simulink model "closed_loop2_simulink"  (R2021b)
settings: Solver=VariableStepAuto  StartTime=0.0  StopTime=15  RelTol=1e-3
values from neighbouring files (symbols this model uses):
  C = I4(1:2,:)    [open_loop.m]
  D = zeros(2,1)    [open_loop.m]
undefined symbols (not defined in the file or in its folder): A, alfa, B, beta, K, sigma_theta, sigma_x, Ts
settings Model: Creator=pieter  LastModifiedBy=pieter

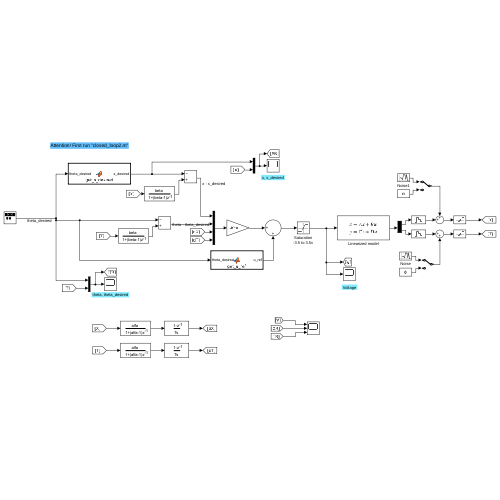
[thumbnail: Simulink's stored preview of the top-level diagram]
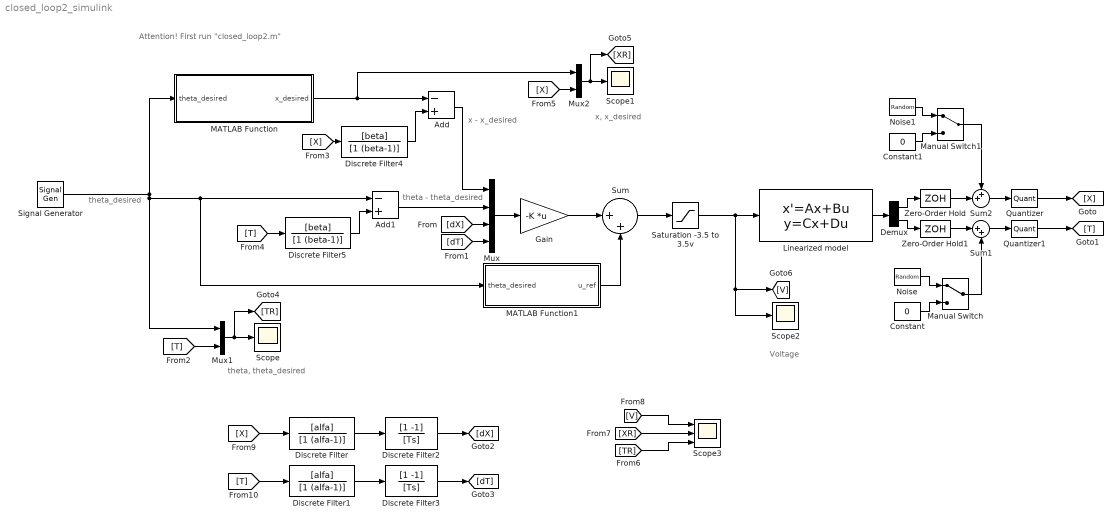
== system closed_loop2_simulink ==
  note: theta - theta_desired
  note: Attention! First run "closed_loop2.m"
  note: Voltage
  note: x - x_desired
  note: x, x_desired
  note: theta, theta_desired
  note: theta_desired
  Add : Sum  Inputs=-+
  Add1 : Sum  Inputs=-+
  Constant : Constant  Value=0
  Constant1 : Constant  Value=0
  Demux : Demux  Outputs=2
  Discrete Filter : DiscreteFilter  Numerator=[alfa]  Denominator=[1 (alfa-1)]
  Discrete Filter1 : DiscreteFilter  Numerator=[alfa]  Denominator=[1 (alfa-1)]
  Discrete Filter2 : DiscreteFilter  Numerator=[1 -1]  Denominator=[Ts]
  Discrete Filter3 : DiscreteFilter  Numerator=[1 -1]  Denominator=[Ts]
  Discrete Filter4 : DiscreteFilter  Numerator=[beta]  Denominator=[1 (beta-1)]
  Discrete Filter5 : DiscreteFilter  Numerator=[beta]  Denominator=[1 (beta-1)]
  Gain : Gain  Gain=-K  Multiplication=Matrix(K*u)
  Linearized model : StateSpace  A=A  B=B  C=C  D=D  InitialCondition=0
  MATLAB Function : MATLAB Function  TreatAsAtomicUnit=on
  MATLAB Function1 : MATLAB Function  TreatAsAtomicUnit=on
  Manual Switch : ManualSwitch
  Manual Switch1 : ManualSwitch
  Mux : Mux
  Mux1 : Mux  Inputs=2
  Mux2 : Mux  Inputs=2
  Noise : RandomNumber  Variance=sigma_theta*sigma_theta  Seed=1  SampleTime=Ts
  Noise1 : RandomNumber  Variance=sigma_x*sigma_x  SampleTime=Ts
  Quantizer : Quantizer  QuantizationInterval=xq  LinearizeAsGain=off
  Quantizer1 : Quantizer  QuantizationInterval=thetaq  LinearizeAsGain=off
  Saturation -3.5 to 3.5v : Saturate  UpperLimit=3.5  LowerLimit=-3.5
  Scope : Scope
  Scope1 : Scope
  Scope2 : Scope
  Scope3 : Scope  NumInputPorts=3
  Signal Generator : SignalGenerator  WaveForm=square  Amplitude=pi/180*2  Frequency=.10
  Sum : Sum  Inputs=|++
  Sum1 : Sum  Inputs=|++
  Sum2 : Sum  Inputs=++|
  Zero-Order Hold : ZeroOrderHold  SampleTime=Ts
  Zero-Order Hold1 : ZeroOrderHold  SampleTime=Ts
  wires:
  Gain/1 -> Sum/1
  [dX] -> Mux/3
  [X] -> Mux2/2
  Signal Generator/1 -> Mux1/1, MATLAB Function1/1(theta_desired), Add1/1, MATLAB Function/1(theta_desired)
  Mux2/1 -> [XR], Scope1/1
  [TR] -> Scope3/3
  Sum/1 -> Saturation -3.5 to 3.5v/1
  Mux/1 -> Gain/1
  Add/1 -> Mux/1
  MATLAB Function/1(x_desired) -> Mux2/1, Add/1
  MATLAB Function1/1(u_ref) -> Sum/2
  [XR] -> Scope3/2
  [T] -> Mux1/2
  Mux1/1 -> [TR], Scope/1
  Add1/1 -> Mux/2
  [dT] -> Mux/4
  [V] -> Scope3/1
  Saturation -3.5 to 3.5v/1 -> Linearized model/1, Scope2/1, [V]
  Constant/1 -> Manual Switch/2
  Noise/1 -> Manual Switch/1
  Constant1/1 -> Manual Switch1/2
  Noise1/1 -> Manual Switch1/1
  Manual Switch/1 -> Sum1/2
  Manual Switch1/1 -> Sum2/1
  Linearized model/1 -> Demux/1
  [X] -> Discrete Filter/1
  [T] -> Discrete Filter1/1
  Discrete Filter/1 -> Discrete Filter2/1
  Discrete Filter1/1 -> Discrete Filter3/1
  Discrete Filter3/1 -> [dT]
  Discrete Filter2/1 -> [dX]
  Demux/1 -> Zero-Order Hold/1
  Demux/2 -> Zero-Order Hold1/1
  Zero-Order Hold1/1 -> Sum1/1
  Zero-Order Hold/1 -> Sum2/2
  Sum2/1 -> Quantizer/1
  Quantizer/1 -> [X]
  Sum1/1 -> Quantizer1/1
  Quantizer1/1 -> [T]
  [X] -> Discrete Filter4/1
  Discrete Filter4/1 -> Add/2
  Discrete Filter5/1 -> Add1/2
  [T] -> Discrete Filter5/1

== matlab function closed_loop2_simulink/MATLAB Function ==
  data: theta_desired input; x_desired output
function x_desired = get_x_desired(theta_desired)
    Mc = 0.52;
    Msw = 3.6;
    Dt = 0.1250;
    Dc = 0.058;
    % From equation (13)
    x_desired = (Mc*Dt+Msw*Dc)*tan(theta_desired)/Mc;
end

== matlab function closed_loop2_simulink/MATLAB Function1 ==
  data: theta_desired input; u_ref output
function u_ref = get_u_ref(theta_desired)
Mc = 0.52;
g = 9.81;
F = Mc*g*sin(theta_desired);
Kt = 0.00767;
Kg = 3.71;
eta_m = 1;
eta_g = 1;
Rm = 2.6;
r = 0.00635;
u_ref = Rm*r/(eta_m*eta_g*Kt*Kg)*F;
